simulink model "DW_MCU_Simulation_Architecture_DualMotor"  (R2018a)
settings: Solver=FixedStepDiscrete  StartTime=0.0  StopTime=20  FixedStep=TimeSteps.ModelStep  RelTol=1e-6
PreLoadFcn:
  | addpath('tools');
  | addpath('tools\Config_UI');
  | addpath('tools\support');
  | addpath('tools\FMIKit_for_Simulink');
  | addpath('tools\FMIKit_for_Simulink\slx');
  | addpath('tools\SpeedCommand');
  | addpath('tools\SpeedCommand\exe');
  | addpath('tools\SpeedCommand\view');
  | addpath('tools\MciAPI');
  | addpath('tools\MciAPI\exe');
  | addpath('tools\MciAPI\exe\enums');
  | addpath('tools\Read_PDB_File');
  | addpath('tools\Read_PDB_File\exe');
  | addpath('tools\PILComm');
  | addpath('tools\PILComm\exe');
  | 
  | addpath('exe');
  | addpath('source\c_code');
  | addpath('source\simulink\PlantModels\Sensor');
  | addpath('source\simulink\PlantModels\Rectifiers');
  | addpath('source\simulink\PlantModels\Motors\CIM');
  | addpath('source\simulink\PlantModels\Motors\BPM');
  | addpath('source\simulink\PlantModels\Motors\BPM\SFunctions\10k\Dyno');
  | addpath('source\simulink\PlantModels\Motors\BPM\SFunctions\10k\HA');
  | addpath('source\simulink\PlantModels\Motors\BPM\SFunctions\10k\VA_Agitation');
  | addpath('source\simulink\PlantModels\Motors\BPM\SFunctions\10k\VA_Spin');
  | addpath('source\simulink\PlantModels\Motors\BPM\SFunctions\16k\Dyno');
  | addpath('source\simulink\PlantModels\Motors\BPM\SFunctions\16k\HA');
  | addpath('source\simulink\PlantModels\Motors\BPM\SFunctions\16k\VA_Agitation');
  | addpath('source\simulink\PlantModels\Motors\BPM\SFunctions\16k\VA_Spin');
  | addpath('source\simulink\PlantModels\Inverter');
  | 
  | 
  | addpath('exported_models');
  | clear all;
  | 
  | try
  | FMIKit.initialize()
  | catch
  | display('FMI Kit Initialization Skipped');
  | end
  | 
  | Sim_Arch_Config_UI_App;
PostLoadFcn:
  | myws = get_param(gcs, 'modelworkspace');
  | myws.clear;
  | clear myws;
  | evalin('base', 'recompile_mcu_sim_arch = 1;');
  | updateModelWS(gcs);
InitFcn:
  | if (evalin('base', 'exist(''smlarch_need_reset'') == 1'))
  |     msgbox('Reload Variables before Running');
  |     set_param(gcs, 'SimulationCommand', 'stop');
  | end
  | BusInit;
  | if(  (exist('SimArchUID')) && (strcmp(SimArchUID, 'a') == 1)  )
  |     updateModelWS(gcs);
  | end
  | useModelWS(gcs);
  | Simulink.sdi.close;
model workspace (MAT data in the model file):
  DC_Bus : struct (value not decoded)
  InputCircuit : struct (value not decoded)
  Mechanical : struct (value not decoded)
  Motor : struct (value not decoded)
  Paths : struct (value not decoded)
  Thermal : struct (value not decoded)
  TimeSteps : struct (value not decoded)
  Variant_Input_Circuit = 5
  Variant_Motor = 3
  Variant_Motor_Control = 1
  Variant_Sensor = 0
  config : struct (value not decoded)
symbols that are objects in the model workspace (value not decoded): DC_Bus, InputCircuit, Motor, Paths, Thermal, TimeSteps
undefined symbols (not defined in the file): DualMotor, Load_D, Load_W, sigbuilder_block, steps
libraries: pdb_libbrowser x7, bpm_dq_S_noH_D_RL_Dyno x2, mciapi_libbrowser x1
(part 2 of 2)

== matlab function DW_MCU_Simulation_Architecture_DualMotor/Signal Processing/Direct  Clark   ==
  data: XAlphaBeta output Bus: XAlphaBetaBus; Xabc input Bus: XabcBus
function XAlphaBeta = DirectClark(Xabc)

XAlphaBeta.Alpha = Xabc.A;
XAlphaBeta.Beta =  sqrt(3)/3*(Xabc.A+2*Xabc.B);

== matlab function DW_MCU_Simulation_Architecture_DualMotor/Motor Coupled With Mechanics/Vpole -> Vphase reconstruction ==
  data: Vpole input Bus: XabcBus size=1; Vout output Bus: XabcBus
function Vout   = Vrec2(Vpole)

Va = Vpole.A;
Vb = Vpole.B;
Vc = Vpole.C;

Vn = (Va + Vb + Vc)/3;

Vphase.A = Va - Vn;
Vphase.B = Vb - Vn;
Vphase.C = Vc - Vn;

Vline.A = Va - Vb;  % Vab
Vline.B = Vb - Vc;  % Vbc
Vline.C = Vc - Va;  % Vca

Vout = Vphase;
end

== matlab function DW_MCU_Simulation_Architecture_DualMotor/DISHWASHER APPLICATION SPECIFIC/MATLAB Function ==
  data: t input; y output int32
function y  = fcn(t)
y = int32(zeros(1,4));
speed = 0;
accel = 0;
load = 0;
trig = 0;


if (t > 2) && (t<3)
    trig = 1;    
elseif (t>=8) && (t<9)
    trig = 1;
elseif (t>=12) && (t<13)
    trig = 1;
end


if (t>=0.5) && (t<4.5)
    speed = 2500;
    accel = 2500;
    load = 1;
elseif (t>=6) && (t<11)
    speed = 0;
    accel = 1500;
    load = 1;
elseif (t>=11) && (t<16)
    speed = 3200;
    accel = 2500;
    load = 0;
end


y(1) = trig;
y(2) = load;
y(3) = speed;
y(4) = accel;

== matlab function DW_MCU_Simulation_Architecture_DualMotor/DISHWASHER APPLICATION SPECIFIC/motorswitch ==
  data: u input; y output
function y = switchfbk(u)
persistent x
if isempty(x)
    x = 0;
end
if u == 0
    y = 1;
else
    y = 0;
end

x = u;

== matlab function DW_MCU_Simulation_Architecture_DualMotor/Simulation Performance/MATLAB Function ==
  data: t input; y output
function y = fcn(t)

persistent t_elaps tval sim_steps t_start t_end
coder.extrinsic('toc') 
coder.extrinsic('tic')
steps_start = 100;%10000;
steps_end = 500;%50000;

if isempty(tval)
    sim_steps = 0;
    tval = uint64(0);
    t_elaps = 0;
    t_start = 0;
    t_end = 0;
end
    
sim_steps = sim_steps +1;

if (sim_steps == steps_start)
    tval = tic;
    t_start = t;
     
end
if (sim_steps == steps_end)
    t_elaps = toc(tval);
    t_end = t;
end
 
if (t_elaps == 0)
    y = 0;
else
    y = t_elaps/(t_end-t_start);
 end

== matlab function DW_MCU_Simulation_Architecture_DualMotor/Signal Processing/Direct Park ==
  data: XAlphaBeta input Bus: XAlphaBetaBus; Xdq output Bus: XdqBus; Theta input
function Xdq = DirectPark(XAlphaBeta,Theta)

Xdq.D  =  XAlphaBeta.Alpha*cos(Theta) + XAlphaBeta.Beta*sin(Theta);
Xdq.Q  = -XAlphaBeta.Alpha*sin(Theta) + XAlphaBeta.Beta*cos(Theta);

== matlab function DW_MCU_Simulation_Architecture_DualMotor/Dual Pump/Vpole -> Vphase reconstruction ==
  data: Vpole input Bus: XabcBus size=1; Vout output Bus: XabcBus
function Vout   = Vrec2(Vpole)

Va = Vpole.A;
Vb = Vpole.B;
Vc = Vpole.C;

Vn = (Va + Vb + Vc)/3;

Vphase.A = Va - Vn;
Vphase.B = Vb - Vn;
Vphase.C = Vc - Vn;

Vline.A = Va - Vb;  % Vab
Vline.B = Vb - Vc;  % Vbc
Vline.C = Vc - Va;  % Vca

Vout = Vphase;
end

== matlab function DW_MCU_Simulation_Architecture_DualMotor/Dual Pump/Vpole -> Vphase reconstruction1 ==
  data: Vpole input Bus: XabcBus size=1; Vout output Bus: XabcBus
function Vout   = Vrec2(Vpole)

Va = Vpole.A;
Vb = Vpole.B;
Vc = Vpole.C;

Vn = (Va + Vb + Vc)/3;

Vphase.A = Va - Vn;
Vphase.B = Vb - Vn;
Vphase.C = Vc - Vn;

Vline.A = Va - Vb;  % Vab
Vline.B = Vb - Vc;  % Vbc
Vline.C = Vc - Va;  % Vca

Vout = Vphase;
end

== matlab function DW_MCU_Simulation_Architecture_DualMotor/Dual Pump/Vpole  switch ==
  data: Vpole_in input Bus: XabcBus size=1; Vpole_Wash output Bus: XabcBus; MotorSwitch input; Vpole_Drain output Bus: XabcBus
function [Vpole_Wash, Vpole_Drain]   = VpoleSwitch(Vpole_in, MotorSwitch)

Wash_Position = 1;

if MotorSwitch == Wash_Position
    Vpole_Wash.A = Vpole_in.A;
    Vpole_Wash.B = Vpole_in.B;
    Vpole_Wash.C = Vpole_in.C;
    Vpole_Drain.A = 0;
    Vpole_Drain.B = 0;
    Vpole_Drain.C = 0;
else
    Vpole_Wash.A = 0;
    Vpole_Wash.B = 0;
    Vpole_Wash.C = 0;
    Vpole_Drain.A = Vpole_in.A;
    Vpole_Drain.B = Vpole_in.B;
    Vpole_Drain.C = Vpole_in.C;
end

== matlab function DW_MCU_Simulation_Architecture_DualMotor/Signal Processing/Direct Park1 ==
  data: XAlphaBeta input Bus: XAlphaBetaBus; Xdq output Bus: XdqBus; Theta input
function Xdq = DirectPark(XAlphaBeta,Theta)

Xdq.D  =  XAlphaBeta.Alpha*cos(Theta) + XAlphaBeta.Beta*sin(Theta);
Xdq.Q  = -XAlphaBeta.Alpha*sin(Theta) + XAlphaBeta.Beta*cos(Theta);

== matlab function DW_MCU_Simulation_Architecture_DualMotor/Dual Pump/Iabc  switch ==
  data: Iabc_Wash input Bus: XabcBus size=1; Power_Wash input; Iabc_Drain input Bus: XabcBus; Power_Drain input; Iabc_out output Bus: XabcBus; MotorSwitch input; Power_out output
function [Iabc_out, Power_out]    = IabcSwitch(Iabc_Wash, Power_Wash, Iabc_Drain, Power_Drain,MotorSwitch)

Wash_Position = 1;

if MotorSwitch == Wash_Position
    Iabc_out.A = Iabc_Wash.A;
    Iabc_out.B = Iabc_Wash.B;
    Iabc_out.C = Iabc_Wash.C;
    Power_out  = Power_Wash;
else
    Iabc_out.A = Iabc_Drain.A;
    Iabc_out.B = Iabc_Drain.B;
    Iabc_out.C = Iabc_Drain.C;
    Power_out  = Power_Drain;
end

== matlab function DW_MCU_Simulation_Architecture_DualMotor/Signal Processing/Vpole -> Vphase reconstruction ==
  data: Vpole input Bus: XabcBus size=1; Vout output Bus: XabcBus
function Vout   = Vrec2(Vpole)

Va = Vpole.A;
Vb = Vpole.B;
Vc = Vpole.C;

Vn = (Va + Vb + Vc)/3;

Vphase.A = Va - Vn;
Vphase.B = Vb - Vn;
Vphase.C = Vc - Vn;

Vline.A = Va - Vb;  % Vab
Vline.B = Vb - Vc;  % Vbc
Vline.C = Vc - Va;  % Vca

Vout = Vphase;
end

== matlab function DW_MCU_Simulation_Architecture_DualMotor/ADC/ADC Raw ==
  data: Iabc input Bus: XabcBus; Iabc_samples output Bus: XabcBus; Vdc input; Vdc_sample output; C1 parameter; C2 parameter; Cvolt parameter; Vcc parameter; ADCBit parameter
function [Iabc_samples, Vdc_sample] = GetADCRawData(Iabc,Vdc, C1, C2, Cvolt, Vcc, ADCBit)
%#codegen


Iabc_samples.A = GetIRaw(Iabc.A,C1,C2,ADCBit, Vcc);
Iabc_samples.B = GetIRaw(Iabc.B,C1,C2,ADCBit,Vcc); 
Iabc_samples.C = GetIRaw(Iabc.C,C1,C2,ADCBit,Vcc); 

Vdc_sample = GetVdcRaw(Vdc,Cvolt,ADCBit,Vcc);
end



function vo = GetIRaw(I,C1,C2,ADCBit,Vcc)
Vout=C1*I+C2;
if(Vout>Vcc)
    Vout=Vcc;
elseif (Vout<0)
        Vout=0;
    end
    vo=round((Vout/Vcc)*2^ADCBit);
end

function vo = GetVdcRaw(Vdc,Cvolt,ADCBit,Vcc)
Vout=Cvolt*Vdc;
if(Vout>Vcc)
    Vout=Vcc;
elseif (Vout<0)
        Vout=0;
    end
    vo=round((Vout/Vcc)*2^ADCBit);
end
